simulink model "B_13"  (R2018b)
settings: Solver=VariableStepAuto  StartTime=0.0  StopTime=1  MaxStep=1e-4  RelTol=1e-6
StopFcn:
  | %CELEC_plot;
settings Model: Creator=Administrator  LastModifiedBy=Administrator

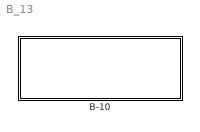
== system B_13 ==
  B-10 : Subsystem  mask{Vset=10, R=2, L=0.02, J=10, KE=1.8, KT=17.2}
      mask prompts: Vset "电源电压(V)"; R "电枢电阻(Ω）"; L "电枢电感(H)"; J "转动惯量(kg.m^3)"; KE "反电势系数(V/rpm)"; KT "电磁转矩系数(N.m/A)"

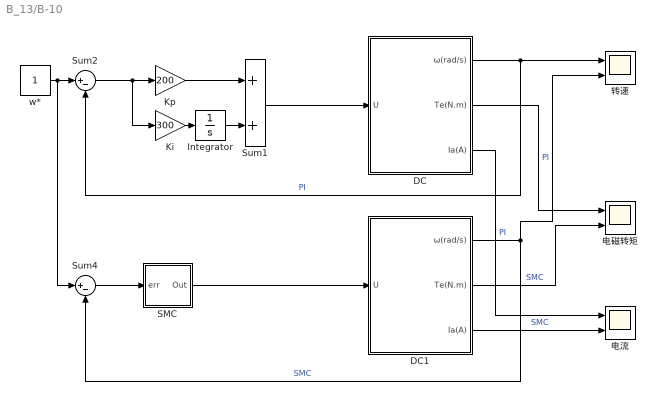
== system B_13/B-10 ==
  DC : Subsystem
  DC1 : Subsystem
  Integrator : Integrator
  Ki : Gain  Gain=300
  Kp : Gain  Gain=200
  SMC : Subsystem  mask{c=500, k=50, e=5, A=1}
      mask prompts: c "增益系数c"; k "增益系数k"; e "增益系数e"; A "增益系数A"
  Sum1 : Sum
  Sum2 : Sum  Inputs=|+-
  Sum4 : Sum  Inputs=|+-
  w* : Constant
  电流 : Scope  NumInputPorts=2
  电磁转矩 : Scope  NumInputPorts=2
  转速 : Scope  NumInputPorts=2
  wires:
  Sum2/1 -> Ki/1, Kp/1
  Kp/1 -> Sum1/1
  Ki/1 -> Integrator/1
  Integrator/1 -> Sum1/2
  w*/1 -> Sum4/1, Sum2/1
  DC/1(ω(rad/s)) -> 转速/1, Sum2/2  "PI"
  Sum1/1 -> DC/1(U)
  DC/2(Te(N.m)) -> 电磁转矩/1  "PI"
  DC/3(Ia(A)) -> 电流/1  "PI"
  SMC/1(Out) -> DC1/1(U)
  DC1/2(Te(N.m)) -> 电磁转矩/2  "SMC"
  DC1/1(ω(rad/s)) -> 转速/2, Sum4/2  "SMC"
  DC1/3(Ia(A)) -> 电流/2  "SMC"
  Sum4/1 -> SMC/1(err)

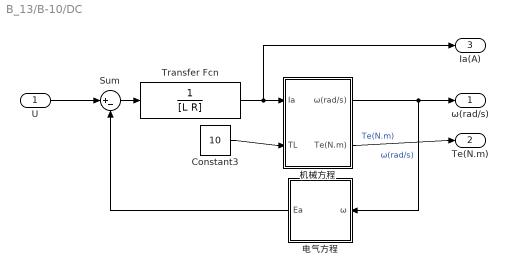
== system B_13/B-10/DC ==
  U : Inport
  Constant3 : Constant  Value=10
  Sum : Sum  Inputs=|+-
  Transfer Fcn : TransferFcn  Denominator=[L R]
  机械方程 : Subsystem
  电气方程 : Subsystem
  ω(rad/s) : Outport
  Te(N.m) : Outport  Port=2
  Ia(A) : Outport  Port=3
  wires:
  Transfer Fcn/1 -> Ia(A)/1, 机械方程/1(Ia)
  Constant3/1 -> 机械方程/2(TL)
  Sum/1 -> Transfer Fcn/1
  机械方程/1(ω(rad/s)) -> 电气方程/1(ω), ω(rad/s)/1  "ω(rad/s)"
  电气方程/1(Ea) -> Sum/2
  U/1 -> Sum/1
  机械方程/2(Te(N.m)) -> Te(N.m)/1  "Te(N.m)"

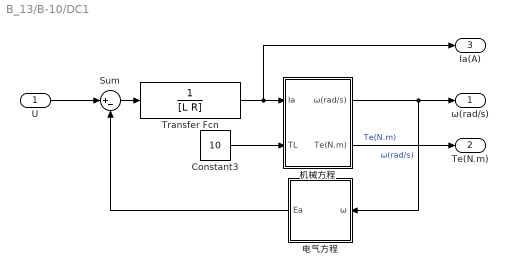
== system B_13/B-10/DC1 ==
  U : Inport
  Constant3 : Constant  Value=10
  Sum : Sum  Inputs=|+-
  Transfer Fcn : TransferFcn  Denominator=[L R]
  机械方程 : Subsystem
  电气方程 : Subsystem
  ω(rad/s) : Outport
  Te(N.m) : Outport  Port=2
  Ia(A) : Outport  Port=3
  wires:
  Transfer Fcn/1 -> Ia(A)/1, 机械方程/1(Ia)
  Constant3/1 -> 机械方程/2(TL)
  Sum/1 -> Transfer Fcn/1
  机械方程/1(ω(rad/s)) -> 电气方程/1(ω), ω(rad/s)/1  "ω(rad/s)"
  电气方程/1(Ea) -> Sum/2
  U/1 -> Sum/1
  机械方程/2(Te(N.m)) -> Te(N.m)/1  "Te(N.m)"

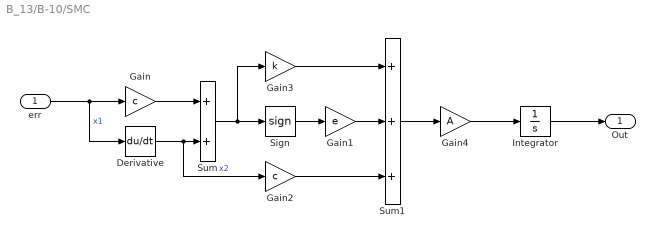
== system B_13/B-10/SMC ==
  err : Inport
  Derivative : Derivative
  Gain : Gain  Gain=c
  Gain1 : Gain  Gain=e
  Gain2 : Gain  Gain=c
  Gain3 : Gain  Gain=k
  Gain4 : Gain  Gain=A
  Integrator : Integrator
  Sign : Signum
  Sum : Sum
  Sum1 : Sum  Inputs=+++
  Out : Outport
  wires:
  Derivative/1 -> Gain2/1, Sum/2  "x2"
  err/1 -> Derivative/1, Gain/1  "x1"
  Gain/1 -> Sum/1
  Sign/1 -> Gain1/1
  Gain1/1 -> Sum1/2
  Gain2/1 -> Sum1/3
  Gain3/1 -> Sum1/1
  Sum/1 -> Gain3/1, Sign/1
  Sum1/1 -> Gain4/1
  Gain4/1 -> Integrator/1
  Integrator/1 -> Out/1

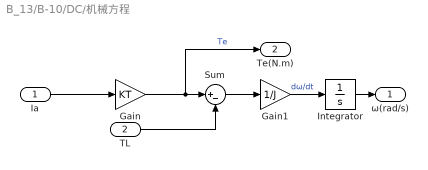
== system B_13/B-10/DC/机械方程 ==
  Ia : Inport
  TL : Inport  Port=2
  Gain : Gain  Gain=KT
  Gain1 : Gain  Gain=1/J
  Integrator : Integrator
  Sum : Sum  Inputs=|+-
  ω(rad/s) : Outport
  Te(N.m) : Outport  Port=2
  wires:
  Gain1/1 -> Integrator/1  "dω/dt"
  Sum/1 -> Gain1/1
  Gain/1 -> Te(N.m)/1, Sum/1  "Te"
  TL/1 -> Sum/2
  Ia/1 -> Gain/1
  Integrator/1 -> ω(rad/s)/1

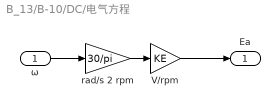
== system B_13/B-10/DC/电气方程 ==
  ω : Inport
  V/rpm : Gain  Gain=KE
  rad/s 2 rpm : Gain  Gain=30/pi
  Ea : Outport
  wires:
  rad/s 2 rpm/1 -> V/rpm/1
  ω/1 -> rad/s 2 rpm/1
  V/rpm/1 -> Ea/1

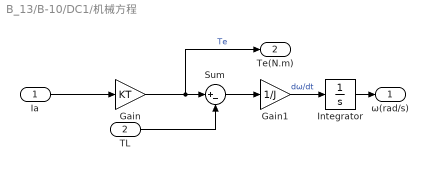
== system B_13/B-10/DC1/机械方程 ==
  Ia : Inport
  TL : Inport  Port=2
  Gain : Gain  Gain=KT
  Gain1 : Gain  Gain=1/J
  Integrator : Integrator
  Sum : Sum  Inputs=|+-
  ω(rad/s) : Outport
  Te(N.m) : Outport  Port=2
  wires:
  Gain1/1 -> Integrator/1  "dω/dt"
  Sum/1 -> Gain1/1
  Gain/1 -> Te(N.m)/1, Sum/1  "Te"
  TL/1 -> Sum/2
  Ia/1 -> Gain/1
  Integrator/1 -> ω(rad/s)/1

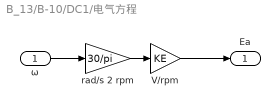
== system B_13/B-10/DC1/电气方程 ==
  ω : Inport
  V/rpm : Gain  Gain=KE
  rad/s 2 rpm : Gain  Gain=30/pi
  Ea : Outport
  wires:
  rad/s 2 rpm/1 -> V/rpm/1
  ω/1 -> rad/s 2 rpm/1
  V/rpm/1 -> Ea/1
